simulink model "TappedDelayLine"  (Simulink 8.6)
settings: Solver=FixedStepDiscrete  StartTime=0  StopTime=inf  RelTol=1e-3
undefined symbols (not defined in the file): gcbh, rcfiltgaincompat
libraries: commchan3 x3, commfilt2 x2, commdigbbndam3 x1, commrandsrc2 x1, simulink x1
CloseFcn:
  | rtwprivate ssgencode ModelCloseRequest Nyquist_Bedingungen
settings Model: Creator=schwall  LastModifiedBy=wunsch
settings DataIOCC: SaveOutput=off  SignalLogging=off  SaveTime=off
settings DebuggingCC: FcnCallInpInsideContextMsg=UseLocalSettings

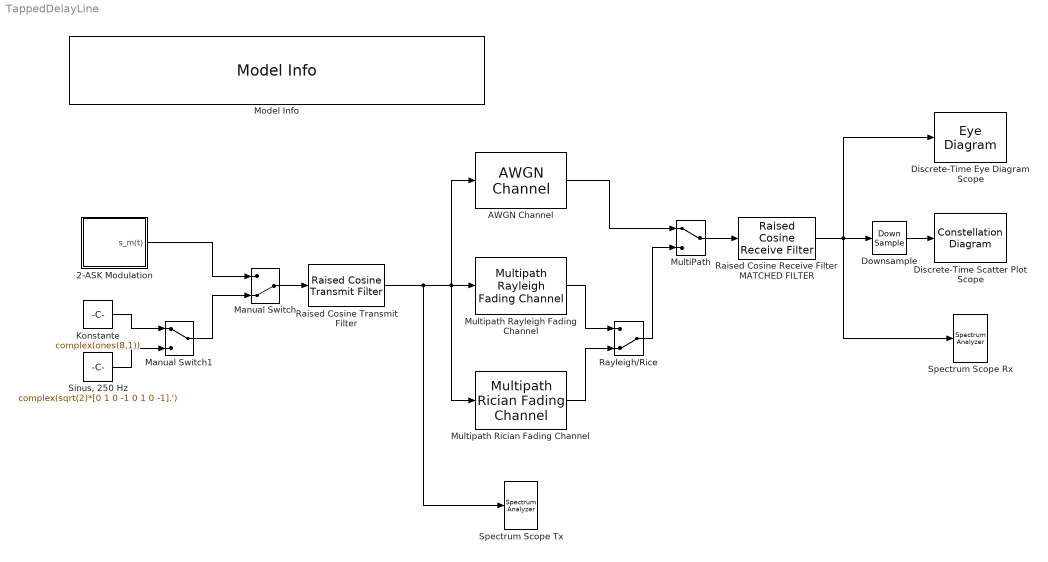
== system TappedDelayLine ==
  2-ASK Modulation : Subsystem
  AWGN Channel : commchan3/AWGN Channel  InputProcessing=Inherited (this choice will be removed - see release notes)  seed=67  noiseMode="Signal to noise ratio  (Es/No)"  EbNodB=10  EsNodB=25  SNRdB=10  bitsPerSym=1  Ps=1/8  Tsym=1/1000  variance=1
  Discrete-Time Eye Diagram Scope : EyeDiagram  Tag=EyeDiagram
  Discrete-Time Scatter Plot Scope : ConstellationDiagram  Tag=ScatterPlot
  Downsample : DownSample  N=8  InputProcessing=Inherited (this choice will be removed - see release notes)  fmode=Maintain input frame rate
  Konstante : Constant  Value=complex(ones(8,1))  VectorParams1D=off
      settings: SamplingMode=Frame based
  Manual Switch : ManualSwitch  CurrentSetting=0
  Manual Switch1 : ManualSwitch
  Model Info : simulink/Model-Wide Utilities/Model Info  BlockCM=None  Frame=on  DisplayStringWithTags=|  HorizontalTextAlignment=Left  LeftAlignmentValue=0.02  SourceBlockDiagram=TappedDelayLine  TagMaxNumber=20
      | Demo Kanalbeschreibung - Tapped Delay Line Modell
      | Vorlesung Nachrichtentechnik II
      | Institut fuer Nachrichtentechnik (CEL)
  MultiPath : ManualSwitch
  Multipath Rayleigh Fading Channel : commchan3/Multipath Rayleigh Fading Channel  maxDopplerShift=200/3.6/3e8*2.4e9  spectrumType=Jakes  sigmaGaussian=1/sqrt(2)  coeffRounded=[1 -1.72 0.785]  freqMinMaxRJakes=[0 1]  freqMinMaxAJakes=[0 1]  sigmaGaussian1=1/sqrt(2)  sigmaGaussian2=1/sqrt(2)  centerFreqGaussian1=0.0  centerFreqGaussian2=0.0  gainGaussian1=0.5  gainGaussian2=0.5  coeffBell=9  dopplerSpectrum=doppler.jakes  pathDelays="[0]     %0.001"  avgPathGaindB=[0]  normalizePathGains=on  seed=73  enableProbe=0  openVisAtStart=off  outPathGains=off  outDelay=off
  Multipath Rician Fading Channel : commchan3/Multipath Rician Fading Channel  K=.1  fdLOS=100  thetaLOS=0  maxDopplerShift=200/3.6/3e8*2.4e9  spectrumType=Jakes  sigmaGaussian=1/sqrt(2)  coeffRounded=[1 -1.72 0.785]  freqMinMaxRJakes=[0 1]  freqMinMaxAJakes=[0 1]  sigmaGaussian1=1/sqrt(2)  sigmaGaussian2=1/sqrt(2)  centerFreqGaussian1=0  centerFreqGaussian2=0  gainGaussian1=0.5  gainGaussian2=0.5  coeffBell=9  dopplerSpectrum=doppler.jakes  pathDelays=[0]  avgPathGaindB=[0]  normalizePathGains=on  seed=73  enableProbe=0  openVisAtStart=off  outPathGains=off  outDelay=off
  Raised Cosine Receive Filter MATCHED FILTER : commfilt2/Raised Cosine Receive Filter  filtType=Square root  N=8  filtSpan=2*(4)  currentFiltSpan=2*(4)  D=4  R=0.2  sampMode=Mute  saveAsFlag=0  rateMode=Downsampling  downFactor=1  downOffset=0  framing=Maintain input frame rate  InputProcessing=Columns as channels (frame based)  checkGain=User-specified  filterGain=(1)*rcfiltgaincompat(gcbh)  checkCoeff=off  variableName=rcRxFilt  launchFVT=off  roundingMode=Floor  overflowMode=off
  Raised Cosine Transmit Filter : commfilt2/Raised Cosine Transmit Filter  filtType=Square root  filtSpan=2*(4)  currentFiltSpan=2*(4)  D=4  R=0.2  sampMode=Mute  saveAsFlag=0  N=8  framing=Maintain input frame rate  InputProcessing=Columns as channels (frame based)  checkGain=User-specified  filterGain=(1)*rcfiltgaincompat(gcbh)  checkCoeff=off  variableName=rcTxFilt  launchFVT=off  roundingMode=Floor  overflowMode=off
  Rayleigh/Rice : ManualSwitch  CurrentSetting=0
  "Sinus, 250 Hz " : Constant  Value=complex(sqrt(2)*[0 1 0 -1 0 1 0 -1].')  VectorParams1D=off
      settings: SamplingMode=Frame based
  Spectrum Scope Rx : SpectrumAnalyzer
  Spectrum Scope Tx : SpectrumAnalyzer
  wires:
  Raised Cosine Transmit Filter/1 -> Spectrum Scope Tx/1, Multipath Rayleigh Fading Channel/1, Multipath Rician Fading Channel/1, AWGN Channel/1
  Raised Cosine Receive Filter MATCHED FILTER/1 -> Spectrum Scope Rx/1, Downsample/1, Discrete-Time Eye Diagram Scope/1
  Manual Switch/1 -> Raised Cosine Transmit Filter/1
  2-ASK Modulation/1(s_m(t)) -> Manual Switch/1
  Downsample/1 -> Discrete-Time Scatter Plot Scope/1
  Konstante/1 -> Manual Switch1/1
  "Sinus, 250 Hz "/1 -> Manual Switch1/2
  Manual Switch1/1 -> Manual Switch/2
  MultiPath/1 -> Raised Cosine Receive Filter MATCHED FILTER/1
  AWGN Channel/1 -> MultiPath/1
  Multipath Rayleigh Fading Channel/1 -> Rayleigh/Rice/1
  Multipath Rician Fading Channel/1 -> Rayleigh/Rice/2
  Rayleigh/Rice/1 -> MultiPath/2

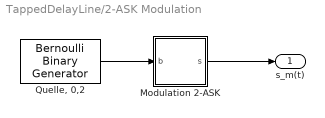
== system TappedDelayLine/2-ASK Modulation ==
  Modulation 2-ASK : Subsystem
  "Quelle, 0,2" : commrandsrc2/Bernoulli Binary Generator  P=0.5  seed=61  Ts=1/1000  frameBased=on  sampPerFrame=8  orient=off  outDataType=double
  s_m(t) : Outport
  wires:
  "Quelle, 0,2"/1 -> Modulation 2-ASK/1(b)
  Modulation 2-ASK/1(s) -> s_m(t)/1

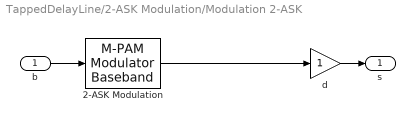
== system TappedDelayLine/2-ASK Modulation/Modulation 2-ASK ==
  b : Inport
  2-ASK Modulation : commdigbbndam3/M-PAM Modulator Baseband  M=2  InType=Integer  Enc=Binary  PowType=Min. distance between symbols  MinDist=2  AvgPow=1  PeakPow=1  outDtype=double  outWordLen=16  outUDDataType=sfix(16)  outFracLenMode=Best precision  outFracLen=15
  d : Gain
  s : Outport
  wires:
  2-ASK Modulation/1 -> d/1
  d/1 -> s/1
  b/1 -> 2-ASK Modulation/1
